simulink model "SS_vs_TF_Simulink"  (R2020a)
settings: Solver=ode4  StartTime=0.0  StopTime=10.0  FixedStep=0.01  RelTol=1e-3
settings Model: Creator=Juan Augusto Paredes  LastModifiedBy=Juan Augusto Paredes

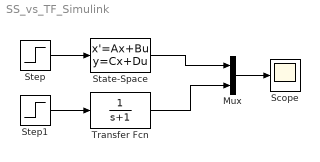
== system SS_vs_TF_Simulink ==
  Mux : Mux  Inputs=2
  Scope : Scope
  State-Space : StateSpace  A=-1  D=0  InitialCondition=2
  Step : Step  After=5  SampleTime=0
  Step1 : Step  After=5  SampleTime=0
  Transfer Fcn : TransferFcn  Denominator=[1 1]
  wires:
  Step/1 -> State-Space/1
  State-Space/1 -> Mux/1
  Step1/1 -> Transfer Fcn/1
  Mux/1 -> Scope/1
  Transfer Fcn/1 -> Mux/2
